simulink model "gggg2"  (R2016b)
settings: Solver=ode4  StartTime=0.0  StopTime=inf  FixedStep=0.002  RelTol=1e-3  EnableMultiTasking=on
values from neighbouring files (symbols this model uses):
  Sxj = [-5.5688169036e-16 5.87476413176e-09 4.69980922027e-08 1.58618466133e-07 3.75984186361e-07 7.34343300515e-07 1.26894350019e-06 2.01503205031e-06 3.00785568581e-06 4.28266054095e-06 5.87469204813e-06 7.81919485707e-06 ... (15001 elements, 1x15001)]    [Sxj.mat]    (also in Sxj10.mat = [-3.2484765271e-16 1.01539136474e-09 8.12312860032e-09 2.741)
  Sxs = [-1.46181443719e-15 1.23369992028e-07 9.86958489185e-07 3.330976688e-06 7.89562117526e-06 1.54210666263e-05 2.66474584787e-05 4.23149056592e-05 6.31634732574e-05 8.9933175228e-05 0.000123363967086 0.000164195738604 ... (15001 elements, 1x15001)]    [Sxs.mat]    (also in Sxs10.mat = [-6.4969530542e-16 8.56736334653e-10 6.85389148561e-09 2.313)
  Vxj = [0 1.76242899492e-05 7.04971163117e-05 0.000158618348628 0.000281987769469 0.000440605074433 0.000634469872145 0.000863581684266 0.00112793994548 0.00142754400352 0.00176239311913 0.00213248646612 ... (15001 elements, 1x15001)]    [Vxj.mat]    (also in Vxj10.mat = [0 3.04617391933e-06 1.21846923369e-05 2.74155452322e-05 4.8)
  Vxs = [0 0.00037010986064 0.00148043578972 0.00333096682877 0.0059216847138 0.00925256387545 0.0133235714393 0.0181346672262 0.0236858037525 0.0299769262308 0.0370079725701 0.044778873377 ... (15001 elements, 1x15001)]    [Vxs.mat]    (also in Vxs10.mat = [0 2.57020934669e-06 1.0280835804e-05 2.31318746131e-05 4.11)
undefined symbols (not defined in the file or in its folder): bit, Standard
libraries: slrtlib x4, slrtsoftinglib x4, simulink x3, dsparch4 x2
settings Model: SimulationMode=external  Creator=Administrator  LastModifiedBy=Tao
settings SolverCC: EnableConcurrentExecution=on
settings DataIOCC: SaveFormat=StructureWithTime
settings OptimizationCC: BlockReduction=off  OptimizeBlockIOStorage=off  BufferReuse=off  GlobalBufferReuse=off  ExpressionFolding=off  LocalBlockOutputs=off
settings HardwareCC: ProdBitPerPointer=32  ProdBitPerSizeT=32  ProdBitPerPtrDiffT=32  ProdLargestAtomicFloat=None  ProdWordSize=32  ProdLongLongMode=on  ProdHWDeviceType=Generic->32-bit x86 compatible
settings RTWCC: SystemTargetFile=slrt.tlc  TemplateMakefile=slrt_default_tmf  Description=Simulink Real-Time  RTWCompilerOptimization=on

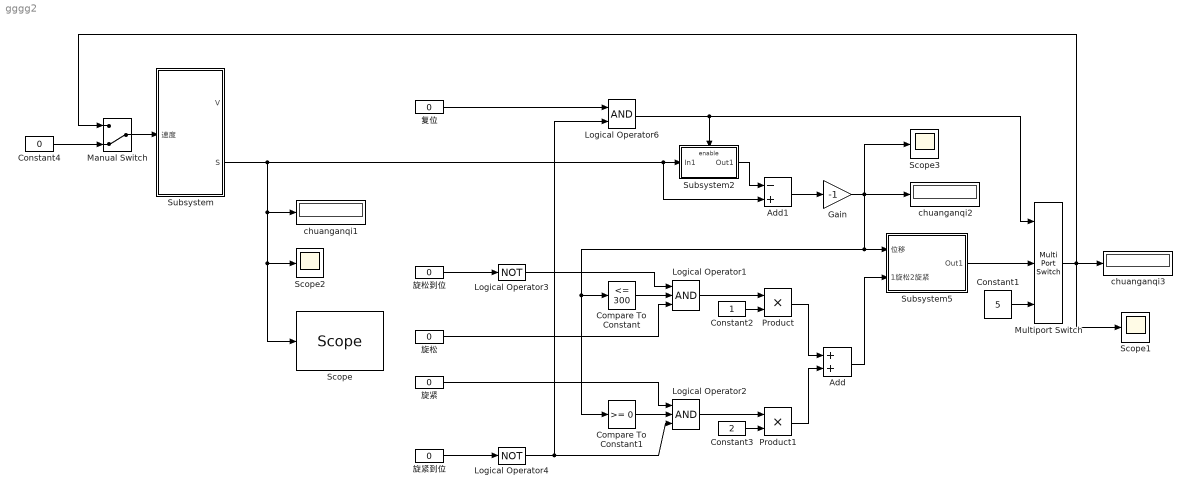
== system gggg2 ==
  Add : Sum
  Add1 : Sum  Inputs=-+
  Compare To Constant : simulink/Logic and Bit Operations/Compare To Constant  relop=<=  const=300  OutDataTypeStr=boolean
  Compare To Constant1 : simulink/Logic and Bit Operations/Compare To Constant  relop=>=  const=0  OutDataTypeStr=boolean
  Constant1 : Constant  Value=5
  Constant2 : Constant
  Constant3 : Constant  Value=2
  Constant4 : Constant  Value=0
  Gain : Gain  Gain=-1
  Logical Operator1 : Logic  Inputs=3  AllPortsSameDT=off  OutDataTypeStr=boolean
  Logical Operator2 : Logic  Inputs=3  AllPortsSameDT=off  OutDataTypeStr=boolean
  Logical Operator3 : Logic  Operator=NOT  AllPortsSameDT=off  OutDataTypeStr=boolean
  Logical Operator4 : Logic  Operator=NOT  AllPortsSameDT=off  OutDataTypeStr=boolean
  Logical Operator6 : Logic  AllPortsSameDT=off  OutDataTypeStr=boolean
  Manual Switch : ManualSwitch  CurrentSetting=0
  Multiport Switch : MultiPortSwitch  DataPortOrder=Zero-based contiguous  Inputs=2
  Product : Product
  Product1 : Product
  "Scope " : slrtlib/Displays and Logging/Scope   scopeno=1  scopetype=Target  autostart=on  viewmode=Graphical redraw  formatstr='%15.6f'  grid=on  ylimits=[0,0]  nosamples=250  noprepostsamples=0  interleave=1  triggermode=FreeRun  triggersignal=1  trigsignalfromport=off  triggerlevel=0.0  triggerslope=Either  triggerscope=1  triggersample=0  filename=data.dat  mode=Lazy  writesize=512  autorestart=off  dynamicfilemode=off  maxwritefilesize=512*1024^2
  Scope1 : Scope
  Scope2 : Scope
  Scope3 : Scope
  Subsystem : Subsystem
  Subsystem2 : Subsystem
  Subsystem5 : Subsystem
  chuanganqi1 : Display
  chuanganqi2 : Display
  chuanganqi3 : Display
  复位 : Constant  Value=0
      settings: OpenFcn=|
      | if get_param(gcb,'value')=='1',
      | set_param(gcb,'value','0');
      | else
      | set_param(gcb,'value','1');end
  旋松 : Constant  Value=0
      settings: OpenFcn=|
      | if get_param(gcb,'value')=='1',
      | set_param(gcb,'value','0');
      | else
      | set_param(gcb,'value','1');end
  旋松到位 : Constant  Value=0
      settings: OpenFcn=|
      | if get_param(gcb,'value')=='1',
      | set_param(gcb,'value','0');
      | else
      | set_param(gcb,'value','1');end
  旋紧 : Constant  Value=0
      settings: OpenFcn=|
      | if get_param(gcb,'value')=='1',
      | set_param(gcb,'value','0');
      | else
      | set_param(gcb,'value','1');end
  旋紧到位 : Constant  Value=0
      settings: OpenFcn=|
      | if get_param(gcb,'value')=='1',
      | set_param(gcb,'value','0');
      | else
      | set_param(gcb,'value','1');end
  wires:
  旋紧/1 -> Logical Operator2/1
  旋松/1 -> Logical Operator1/3
  Subsystem/2(S) -> Add1/2, Subsystem2/1(In1), "Scope "/1, Scope2/1, chuanganqi1/1
  Add/1 -> Subsystem5/2(1旋松2旋紧)
  Compare To Constant/1 -> Logical Operator1/2
  Logical Operator1/1 -> Product/1
  Compare To Constant1/1 -> Logical Operator2/2
  旋松到位/1 -> Logical Operator3/1
  旋紧到位/1 -> Logical Operator4/1
  Logical Operator3/1 -> Logical Operator1/1
  Logical Operator4/1 -> Logical Operator6/2, Logical Operator2/3
  Logical Operator6/1 -> Subsystem2/Enable, Multiport Switch/1
  Subsystem2/1(Out1) -> Add1/1
  Subsystem5/1(Out1) -> Multiport Switch/2
  Constant1/1 -> Multiport Switch/3
  复位/1 -> Logical Operator6/1
  Add1/1 -> Gain/1
  Constant2/1 -> Product/2
  Product/1 -> Add/1
  Constant3/1 -> Product1/2
  Logical Operator2/1 -> Product1/1
  Product1/1 -> Add/2
  Gain/1 -> Scope3/1, chuanganqi2/1, Compare To Constant1/1, Compare To Constant/1, Subsystem5/1(位移)
  Multiport Switch/1 -> Manual Switch/1, Scope1/1, chuanganqi3/1
  Constant4/1 -> Manual Switch/2
  Manual Switch/1 -> Subsystem/1(速度)

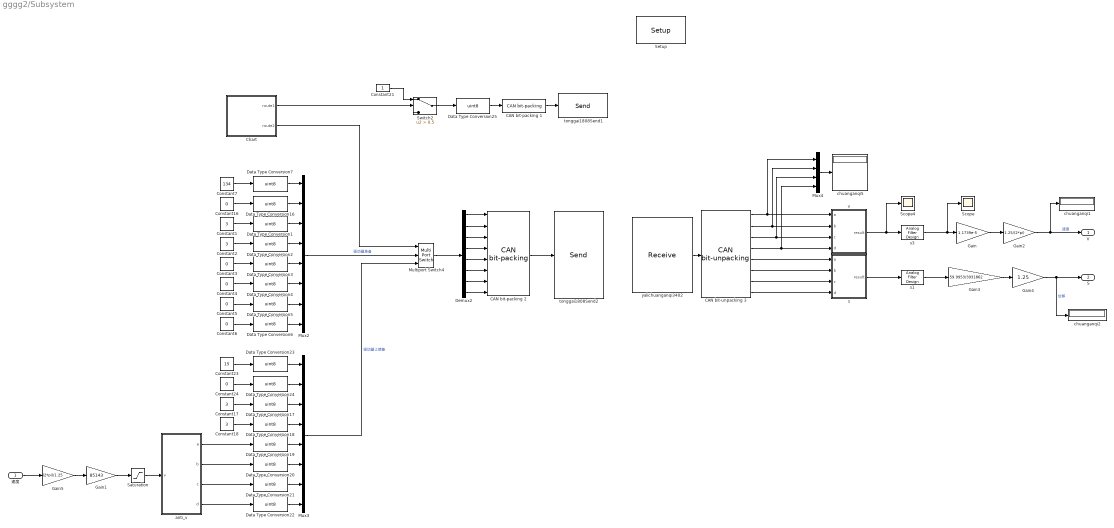
== system gggg2/Subsystem ==
  速度 : Inport
  CAN bit-packing 1 : slrtlib/CAN/Utilities/CAN bit-packing   bitpatterns={[0:7]}
  CAN bit-packing 2 : slrtlib/CAN/Utilities/CAN bit-packing   bitpatterns={ [0:7] [8:15] [16:23] [24:31] [32:39] [40:47] [48:55] [56:63]}
  CAN bit-unpacking 3 : slrtlib/CAN/Utilities/CAN bit-unpacking   bitpatterns={ [0:7] [8:15] [16:23] [24:31] [32:39] [40:47] [48:55] [56:63]}  dtypes={ 'uint8','uint8','uint8','uint8' ,'uint8','uint8','uint8','uint8'}
  Chart : Stateflow chart  TreatAsAtomicUnit=on
  Constant{1..2,17..18} (4 alike) : Constant  Value=3
  Constant{3..6,16,24} (6 alike) : Constant  Value=0
  Constant21 : Constant
  Constant23 : Constant  Value=15
  Constant7 : Constant  Value=134
  Data Type Conversion{1..7,16..25} (17 alike) : DataTypeConversion  OutDataTypeStr=uint8
  Demux2 : Demux  Outputs=8
  Gain : Gain  Gain=1.1739e-5
  Gain1 : Gain  Gain=85143
  Gain2 : Gain  Gain=1.25/(2*pi)
  Gain3 : Gain  Gain=59.9953/3931862
  Gain4 : Gain  Gain=1.25
  Gain5 : Gain  Gain=(2*pi)/1.25
  Multiport Switch4 : MultiPortSwitch  DataPortOrder=Zero-based contiguous  Inputs=2
  Mux2 : Mux  Inputs=8
  Mux3 : Mux  Inputs=8
  Mux4 : Mux
  Saturation : Saturate  UpperLimit=2147483647  LowerLimit=-2147483647
  Scope : Scope
  Scope4 : Scope
  "Setup " : slrtsoftinglib/CAN-AC2-PCI SJA 1000/Setup   board=1  can1bus=Highspeed (ISO 11898)  can1Baudrate=1 MBaud  can1UserBR=[1,1,4,3]  can2bus=Highspeed (ISO 11898)  can2Baudrate=1 MBaud  can2UserBR=[1,1,4,3]  init=[]  term=[]  bus_off_out=off  bus_off_rec=Off  ioBaseAddress=-1
  Switch2 : Switch  Criteria=u2 > Threshold  Threshold=0.5
  anti_v : MATLAB Function  TreatAsAtomicUnit=on
  chuanganqi1 : Display
  chuanganqi2 : Display
  chuanganqi5 : Display
  s : MATLAB Function  TreatAsAtomicUnit=on
  s1 : dsparch4/Analog Filter Design  method=Butterworth  filttype=Lowpass  N=1  Wlo=10  Whi=80  Rp=2  Rs=40
  s3 : dsparch4/Analog Filter Design  method=Butterworth  filttype=Lowpass  N=1  Wlo=10  Whi=80  Rp=2  Rs=40
  tonggai1808Send1 : slrtsoftinglib/CAN-AC2-PCI SJA 1000/Send   board=1  canPort=CAN 2  range=Standard (11-bit)  ids=0  sizes=[8]  output=off  ts=-1  ididx=[0]
  tonggai1808Send2 : slrtsoftinglib/CAN-AC2-PCI SJA 1000/Send   board=1  canPort=CAN 2  range=Standard (11-bit)  ids=1537  sizes=[8]  output=off  ts=-1  ididx=[0]
  v : MATLAB Function  TreatAsAtomicUnit=on
  yalichuanganqi3402 : slrtsoftinglib/CAN-AC2-PCI SJA 1000/Receive   board=1  canPort=CAN 2  range=Standard (11-bit)  ids=385  lengths=8  output=Data  inten=off  ts=-1  ididx=[0]
  V : Outport
  S : Outport  Port=2
  wires:
  Data Type Conversion4/1 -> Mux2/6
  Constant6/1 -> Data Type Conversion6/1
  Constant2/1 -> Data Type Conversion2/1
  Constant16/1 -> Data Type Conversion16/1
  Data Type Conversion6/1 -> Mux2/8
  Data Type Conversion1/1 -> Mux2/3
  Data Type Conversion16/1 -> Mux2/2
  Constant7/1 -> Data Type Conversion7/1
  Constant1/1 -> Data Type Conversion1/1
  Data Type Conversion2/1 -> Mux2/4
  Constant5/1 -> Data Type Conversion5/1
  Data Type Conversion23/1 -> Mux3/1
  Data Type Conversion7/1 -> Mux2/1
  Data Type Conversion5/1 -> Mux2/7
  Constant4/1 -> Data Type Conversion4/1
  Data Type Conversion3/1 -> Mux2/5
  Data Type Conversion22/1 -> Mux3/8
  Constant18/1 -> Data Type Conversion18/1
  Demux2/3 -> CAN bit-packing 2/3
  Demux2/7 -> CAN bit-packing 2/7
  anti_v/2(b) -> Data Type Conversion20/1
  Data Type Conversion20/1 -> Mux3/6
  Data Type Conversion19/1 -> Mux3/5
  anti_v/1(a) -> Data Type Conversion19/1
  Constant24/1 -> Data Type Conversion24/1
  Demux2/8 -> CAN bit-packing 2/8
  Constant23/1 -> Data Type Conversion23/1
  Constant17/1 -> Data Type Conversion17/1
  Data Type Conversion17/1 -> Mux3/3
  Data Type Conversion24/1 -> Mux3/2
  Data Type Conversion21/1 -> Mux3/7
  Gain1/1 -> Saturation/1
  anti_v/4(d) -> Data Type Conversion22/1
  Data Type Conversion18/1 -> Mux3/4
  Demux2/1 -> CAN bit-packing 2/1
  anti_v/3(c) -> Data Type Conversion21/1
  Saturation/1 -> anti_v/1(v)
  Demux2/2 -> CAN bit-packing 2/2
  Demux2/4 -> CAN bit-packing 2/4
  Demux2/5 -> CAN bit-packing 2/5
  Demux2/6 -> CAN bit-packing 2/6
  Multiport Switch4/1 -> Demux2/1
  Mux3/1 -> Multiport Switch4/3  "驱动器上使能"
  CAN bit-packing 2/1 -> tonggai1808Send2/1
  Mux2/1 -> Multiport Switch4/2  "驱动器准备"
  Gain4/1 -> S/1, chuanganqi2/1  "位移"
  yalichuanganqi3402/1 -> CAN bit-unpacking 3/1
  CAN bit-unpacking 3/4 -> Mux4/4, v/4(d)
  CAN bit-unpacking 3/2 -> v/2(b), Mux4/2
  Mux4/1 -> chuanganqi5/1
  Gain/1 -> Gain2/1
  CAN bit-unpacking 3/1 -> v/1(a), Mux4/1
  CAN bit-unpacking 3/3 -> v/3(c), Mux4/3
  s3/1 -> Scope/1, Gain/1
  v/1(result) -> Scope4/1, s3/1
  Gain3/1 -> Gain4/1
  Gain2/1 -> V/1, chuanganqi1/1  "速度"
  Gain5/1 -> Gain1/1
  CAN bit-packing 1/1 -> tonggai1808Send1/1
  Data Type Conversion25/1 -> CAN bit-packing 1/1
  Switch2/1 -> Data Type Conversion25/1
  Constant21/1 -> Switch2/1
  Constant3/1 -> Data Type Conversion3/1
  CAN bit-unpacking 3/5 -> s/1(a)
  CAN bit-unpacking 3/6 -> s/2(b)
  CAN bit-unpacking 3/7 -> s/3(c)
  CAN bit-unpacking 3/8 -> s/4(d)
  s1/1 -> Gain3/1
  s/1(result) -> s1/1
  速度/1 -> Gain5/1
  Chart/2(route2) -> Multiport Switch4/1
  Chart/1(route1) -> Switch2/2

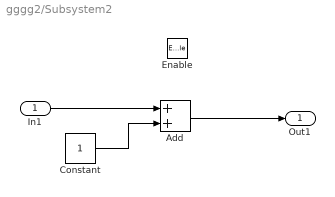
== system gggg2/Subsystem2 ==
  In1 : Inport
  Enable : EnablePort
  Add : Sum
  Constant : Constant
  Out1 : Outport
  wires:
  In1/1 -> Add/1
  Add/1 -> Out1/1
  Constant/1 -> Add/2

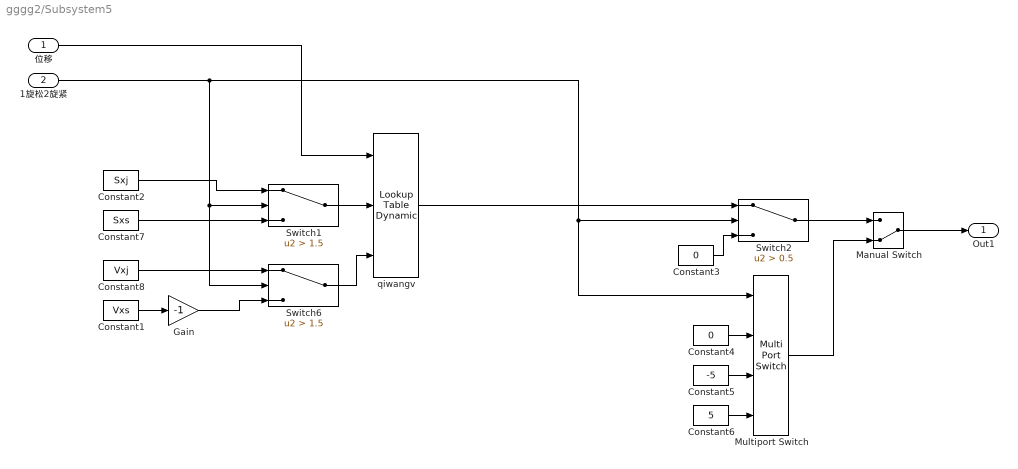
== system gggg2/Subsystem5 ==
  位移 : Inport
  1旋松2旋紧 : Inport  Port=2
  Constant1 : Constant  Value=Vxs
  Constant2 : Constant  Value=Sxj
  Constant3 : Constant  Value=0
  Constant4 : Constant  Value=0
  Constant5 : Constant  Value=-5
  Constant6 : Constant  Value=5
  Constant7 : Constant  Value=Sxs
  Constant8 : Constant  Value=Vxj
  Gain : Gain  Gain=-1
  Manual Switch : ManualSwitch  CurrentSetting=0
  Multiport Switch : MultiPortSwitch  DataPortOrder=Zero-based contiguous
  Switch1 : Switch  Criteria=u2 > Threshold  Threshold=1.5
  Switch2 : Switch  Criteria=u2 > Threshold  Threshold=0.5
  Switch6 : Switch  Criteria=u2 > Threshold  Threshold=1.5
  qiwangv : simulink/Lookup Tables/Lookup Table Dynamic  LookUpMeth=Interpolation-Use End Values  OutDataType=float('double')  OutScaling=[]  OutputDataTypeScalingMode=Specify via dialog  OutDataTypeStr=float('double')  DoSatur=off
  Out1 : Outport
  wires:
  1旋松2旋紧/1 -> Switch2/2, Multiport Switch/1, Switch6/2, Switch1/2
  Constant7/1 -> Switch1/3
  Constant1/1 -> Gain/1
  Switch6/1 -> qiwangv/3
  Constant8/1 -> Switch6/1
  Constant2/1 -> Switch1/1
  Switch1/1 -> qiwangv/2
  位移/1 -> qiwangv/1
  Switch2/1 -> Manual Switch/1
  Constant3/1 -> Switch2/3
  Gain/1 -> Switch6/3
  qiwangv/1 -> Switch2/1
  Constant4/1 -> Multiport Switch/2
  Constant5/1 -> Multiport Switch/3
  Constant6/1 -> Multiport Switch/4
  Manual Switch/1 -> Out1/1
  Multiport Switch/1 -> Manual Switch/2

== matlab function gggg2/Subsystem/anti_v ==
  data: v input; a output; b output; c output; d output
function [a, b, c, d]  = anti_velocity(v)
if v>=0
    BASE = '00000000000000000000000000000000';%一共32位
    Vbin = dec2bin(v);
    LVbin = length(Vbin);
    for i = 1:LVbin
        BASE(32-LVbin+i) = Vbin(i);
    end
    Vbin = BASE;
else
    BASE = '00000000000000000000000000000000';%一共32位
    V = 4294967295 + v + 1; %bin2dec('11111111111111111111111111111111')（一共32位）=4294967295
    Vbin = dec2bin(V);
    LVbin = length(Vbin);
    for i = 1:LVbin
        BASE(32-LVbin+i) = Vbin(i);
    end
    Vbin = BASE;
end
D = Vbin(1:8);
C = Vbin(9:16);
B = Vbin(17:24);
A = Vbin(25:32);
d = bin2dec(D);
c = bin2dec(C);
b = bin2dec(B);
a = bin2dec(A);
end

== matlab function gggg2/Subsystem/v ==
  data: a input; result output; b input; c input; d input
function result  = conversion(a, b, c, d)
A = dec2bin(a);
B = dec2bin(b);
C = dec2bin(c);
D = dec2bin(d);

BASE = '00000000';
LA = length(A);
for i = 1:LA
    BASE(8-LA+i) = A(i);
end
A = BASE;

BASE = '00000000';
LB = length(B);
for i = 1:LB
    BASE(8-LB+i) = B(i);
end
B = BASE;

BASE = '00000000';
LC = length(C);
for i = 1:LC
    BASE(8-LC+i) = C(i);
end
C = BASE;

BASE = '00000000';
LD = length(D);
for i = 1:LD
    BASE(8-LD+i) = D(i);
end
D = BASE;

Vbin = [D, C, B, A];
R = bin2dec(Vbin);
if d < 128  %bin2dec('10000000')=128
    result = R;
else
    R = R-1;
    result = -(4294967295 - R); %bin2dec('11111111111111111111111111111111')（一共32位）=4294967295
end

== matlab function gggg2/Subsystem/s ==
  data: a input; result output; b input; c input; d input
function result  = conversion(a, b, c, d)
A = dec2bin(a);
B = dec2bin(b);
C = dec2bin(c);
D = dec2bin(d);

BASE = '00000000';
LA = length(A);
for i = 1:LA
    BASE(8-LA+i) = A(i);
end
A = BASE;

BASE = '00000000';
LB = length(B);
for i = 1:LB
    BASE(8-LB+i) = B(i);
end
B = BASE;

BASE = '00000000';
LC = length(C);
for i = 1:LC
    BASE(8-LC+i) = C(i);
end
C = BASE;

BASE = '00000000';
LD = length(D);
for i = 1:LD
    BASE(8-LD+i) = D(i);
end
D = BASE;

Vbin = [D, C, B, A];
R = bin2dec(Vbin);
if d < 128  %bin2dec('10000000')=128
    result = R;
else
    R = R-1;
    result = -(4294967295 - R); %bin2dec('11111111111111111111111111111111')（一共32位）=4294967295
end

== stateflow chart gggg2/Subsystem/Chart ==
  state route
    state on1
      en:
      route1=1;
      route2=0;
    state on3
      en:
      route1=0;
      route2=1;
    state on4
      en:
      route1=0;
      route2=2;
    (default) -> on1
    on1 -> on3 : after(5,tick)
    on3 -> on4 : after(10,tick)
  data: route1 output; route2 output
